simulink model "simulink_test"  (R2016b)
settings: Solver=VariableStepAuto  StartTime=0.0  StopTime=T  RelTol=1e-3
values from neighbouring files (symbols this model uses):
  A = [-R1/L1 0 0 -1/L1 ... (first row only)    [h1.m]    (also in h1_test.m = [-R1/Lt1 0 0 -1/Lt1)
  Atilde = 1000    [h1.m]    (also in h1_test.m)
  B = [1/L1 0 ... (first row only)    [h1.m]    (also in h1_test.m = [1/Lt1 0)
  C = [0 0 0 1]    [h1.m]    (also in h1_test.m)
  D = [0 0]    [h1.m]    (also in h1_test.m)
  ftilde = 5    [h1.m]    (also in h1_test.m)
settings Model: Creator=rickardandersson  LastModifiedBy=rickardandersson

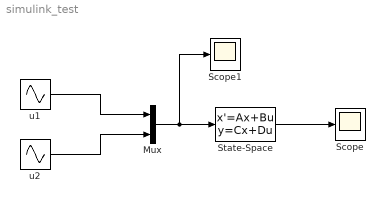
== system simulink_test ==
  Mux : Mux  Inputs=2
  Scope : Scope
  Scope1 : Scope
  State-Space : StateSpace  A=A  B=B  C=C  D=D  X0=[0,0,0,6e3]
  "u1 " : Sin  Amplitude=Atilde  Frequency=2*pi*ftilde  SampleTime=0
  u2 : Sin  Amplitude=Atilde  Frequency=2*pi*ftilde  Phase=pi/2  SampleTime=0
  wires:
  Mux/1 -> Scope1/1, State-Space/1
  State-Space/1 -> Scope/1
  "u1 "/1 -> Mux/1
  u2/1 -> Mux/2
